simulink model "ball_bouncing_v2"  (R2017b)
settings: Solver=FixedStepAuto  StartTime=0.0  StopTime=0.001  FixedStep=0.0001  RelTol=1e-3
settings Model: Creator=Vincent  LastModifiedBy=Vincent
settings SolverCC: AlgebraicLoopSolver=LineSearch

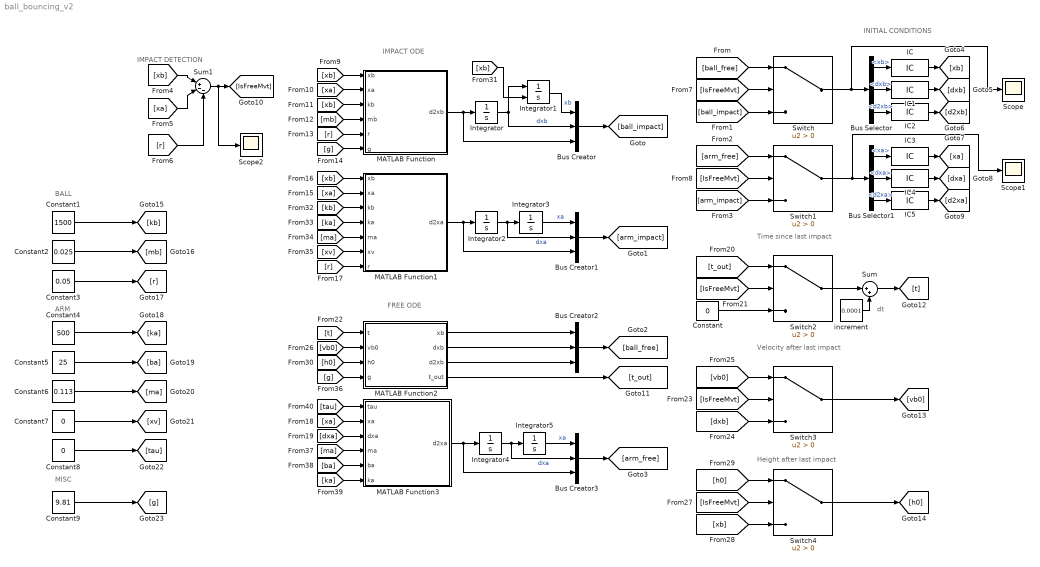
== system ball_bouncing_v2 ==
  note: dt
  note: MISC
  note: BALL
  note: INITIAL CONDITIONS
  note: Time since last impact
  note: IMPACT DETECTION
  note: FREE ODE
  note: IMPACT ODE
  note: Velocity after last impact
  note: Height after last impact
  note: ARM
  Bus Creator{,1..3} (4 alike) : BusCreator  Inputs=3
  Bus Selector : BusSelector  OutputSignals=xb,dxb,d2xb
  Bus Selector1 : BusSelector  OutputSignals=xa,dxa,d2xa
  Constant : Constant  Value=0
  Constant1 : Constant  Value=1500
  Constant2 : Constant  Value=0.025
  Constant3 : Constant  Value=0.05
  Constant4 : Constant  Value=500
  Constant5 : Constant  Value=25
  Constant6 : Constant  Value=0.113
  Constant7 : Constant  Value=0
  Constant8 : Constant  Value=0
  Constant9 : Constant  Value=9.81
  IC : InitialCondition  Value=0.5
  IC{1..5} (5 alike) : InitialCondition  Value=0
  Integrator{,2..5} (5 alike) : Integrator
  Integrator1 : Integrator  InitialConditionSource=external
  MATLAB Function : MATLAB Function  TreatAsAtomicUnit=on
  MATLAB Function1 : MATLAB Function  TreatAsAtomicUnit=on
  MATLAB Function2 : MATLAB Function  TreatAsAtomicUnit=on
  MATLAB Function3 : MATLAB Function  TreatAsAtomicUnit=on
  Scope : Scope
  Scope1 : Scope
  Scope2 : Scope
  Sum : Sum  Inputs=|++
  Sum1 : Sum  Inputs=|+--
  Switch{,1..4} (5 alike) : Switch  Criteria=u2 > Threshold
  increment : Constant  Value=0.0001
  wires:
  MATLAB Function/1(d2xb) -> Bus Creator/3, Integrator/1
  Integrator/1 -> Bus Creator/2, Integrator1/1  "dxb"
  Integrator2/1 -> Bus Creator1/2, Integrator3/1  "dxa"
  MATLAB Function1/1(d2xa) -> Bus Creator1/3, Integrator2/1
  MATLAB Function3/1(d2xa) -> Bus Creator3/3, Integrator4/1
  Integrator4/1 -> Bus Creator3/2, Integrator5/1  "dxa"
  Integrator1/1 -> Bus Creator/1  "xb"
  Integrator3/1 -> Bus Creator1/1  "xa"
  Integrator5/1 -> Bus Creator3/1  "xa"
  MATLAB Function2/2(dxb) -> Bus Creator2/2
  MATLAB Function2/1(xb) -> Bus Creator2/1
  MATLAB Function2/3(d2xb) -> Bus Creator2/3
  Bus Creator/1 -> [ball_impact]
  Bus Creator1/1 -> [arm_impact]
  Bus Creator2/1 -> [ball_free]
  Bus Creator3/1 -> [arm_free]
  [ball_free] -> Switch/1
  [ball_impact] -> Switch/3
  [arm_free] -> Switch1/1
  [arm_impact] -> Switch1/3
  Switch/1 -> Scope/1, Bus Selector/1
  Switch1/1 -> Scope1/1, Bus Selector1/1
  Sum1/1 -> Scope2/1, [IsFreeMvt]
  [xb] -> Sum1/1
  [xa] -> Sum1/2
  [r] -> Sum1/3
  [IsFreeMvt] -> Switch/2
  [IsFreeMvt] -> Switch1/2
  [xb] -> MATLAB Function/1(xb)
  [xa] -> MATLAB Function/2(xa)
  [xb] -> MATLAB Function1/1(xb)
  [xa] -> MATLAB Function1/2(xa)
  [r] -> MATLAB Function1/7(r)
  [xa] -> MATLAB Function3/2(xa)
  [dxa] -> MATLAB Function3/3(dxa)
  [t_out] -> Switch2/1
  [IsFreeMvt] -> Switch2/2
  Constant/1 -> Switch2/3
  MATLAB Function2/4(t_out) -> [t_out]
  Switch2/1 -> Sum/1
  Sum/1 -> [t]
  increment/1 -> Sum/2
  [t] -> MATLAB Function2/1(t)
  [IsFreeMvt] -> Switch3/2
  [dxb] -> Switch3/3
  Switch3/1 -> [vb0]
  [vb0] -> Switch3/1
  [vb0] -> MATLAB Function2/2(vb0)
  [h0] -> Switch4/1
  Switch4/1 -> [h0]
  [xb] -> Switch4/3
  [IsFreeMvt] -> Switch4/2
  [h0] -> MATLAB Function2/3(h0)
  Bus Selector/1 -> IC/1  "<xb>"
  IC/1 -> [xb]
  Bus Selector/2 -> IC1/1  "<dxb>"
  IC1/1 -> [dxb]
  Bus Selector/3 -> IC2/1  "<d2xb>"
  IC2/1 -> [d2xb]
  Bus Selector1/1 -> IC3/1  "<xa>"
  IC3/1 -> [xa]
  Bus Selector1/2 -> IC4/1  "<dxa>"
  IC4/1 -> [dxa]
  Bus Selector1/3 -> IC5/1  "<d2xa>"
  IC5/1 -> [d2xa]
  [xb] -> Integrator1/2
  Constant1/1 -> [kb]
  Constant3/1 -> [r]
  Constant2/1 -> [mb]
  Constant5/1 -> [ba]
  Constant6/1 -> [ma]
  Constant4/1 -> [ka]
  [kb] -> MATLAB Function1/3(kb)
  [ka] -> MATLAB Function1/4(ka)
  [xv] -> MATLAB Function1/6(xv)
  [ma] -> MATLAB Function1/5(ma)
  Constant7/1 -> [xv]
  Constant8/1 -> [tau]
  Constant9/1 -> [g]
  [g] -> MATLAB Function2/4(g)
  [ka] -> MATLAB Function3/6(ka)
  [ba] -> MATLAB Function3/5(ba)
  [ma] -> MATLAB Function3/4(ma)
  [tau] -> MATLAB Function3/1(tau)
  [g] -> MATLAB Function/6(g)
  [r] -> MATLAB Function/5(r)
  [mb] -> MATLAB Function/4(mb)
  [xb] -> MATLAB Function/3(kb)

== matlab function ball_bouncing_v2/MATLAB Function1 ==
  data: xb input; d2xa output; xa input; kb input; ka input; ma input; xv input; r input
function d2xa = d2xa_ode(xb, xa, kb, ka, ma, xv, r)

    d2xa = (-ka*(xa - xv) + kb*(xb - xa - r))/ma;

== matlab function ball_bouncing_v2/MATLAB Function ==
  data: xb input; d2xb output; xa input; kb input; mb input; r input; g input
function d2xb = d2xb_ode(xb, xa, kb, mb, r, g)

    d2xb = (-kb*(xb - xa - r) - mb * g)/mb;

== matlab function ball_bouncing_v2/MATLAB Function2 ==
  data: t input; xb output; vb0 input; h0 input; g input; dxb output; d2xb output; t_out output
function [xb, dxb, d2xb, t_out] = ballistic_eq(t, vb0, h0, g)

    xb = -0.5*g*t^2 + vb0*t + h0;
    dxb = -g*t + vb0;
    d2xb = -g;
    t_out = t;

== matlab function ball_bouncing_v2/MATLAB Function3 ==
  data: tau input; d2xa output; xa input; dxa input; ma input; ba input; ka input
function d2xa = arm_eq(tau, xa, dxa, ma, ba, ka)

    d2xa = (tau - ba * dxa - ka * xa)/ma;
